simulink model "InverseTest"  (R2021a)
settings: Solver=VariableStepAuto  StartTime=0.0  StopTime=50.0  RelTol=1e-3
settings Model: Creator=drak0  LastModifiedBy=drak0

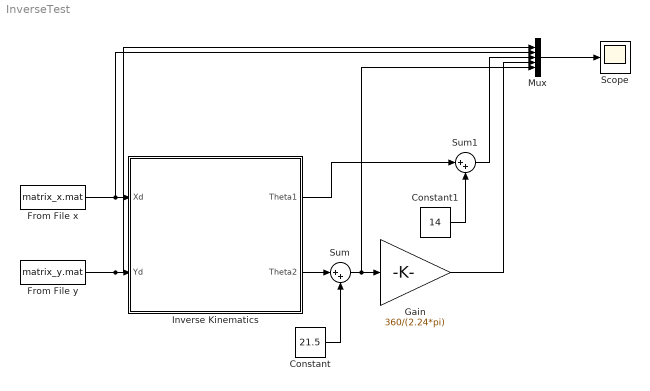
== system InverseTest ==
  Constant : Constant  Value=21.5
  Constant1 : Constant  Value=14
  From File x : FromFile  FileName=matrix_x.mat  SampleTime=0
  From File y : FromFile  FileName=matrix_y.mat  SampleTime=0
  Gain : Gain  Gain=360/(2.24*pi)
  Inverse Kinematics : MATLAB Function  TreatAsAtomicUnit=on
  Mux : Mux  Inputs=5
  Scope : Scope
  Sum : Sum  Inputs=|++
  Sum1 : Sum  Inputs=|++
  wires:
  Mux/1 -> Scope/1
  From File x/1 -> Mux/2, Inverse Kinematics/1(Xd)
  From File y/1 -> Mux/1, Inverse Kinematics/2(Yd)
  Gain/1 -> Mux/4
  Inverse Kinematics/2(Theta2) -> Sum/1
  Sum/1 -> Mux/5, Gain/1
  Constant/1 -> Sum/2
  Inverse Kinematics/1(Theta1) -> Sum1/1
  Constant1/1 -> Sum1/2
  Sum1/1 -> Mux/3

== matlab function InverseTest/Inverse Kinematics ==
  data: Xd input; Theta1 output; Yd input; Theta2 output
function [Theta1,Theta2] = InverseKinematics(Xd,Yd)
l1 = 2.25;
l2 = 21.5;
q1r = (atan2((sqrt(abs(-l1^2+Xd^2+Yd^2))+Yd),(l1+Xd)));
Theta1 = rad2deg(q1r);
Theta2 = -sin(q1r)*Xd +cos(q1r)*Yd-l2;
